simulink model "ROBOT_OK"  (R2021a)
settings: Solver=FixedStepAuto  StartTime=0.0  StopTime=inf  FixedStep=0.001  RelTol=1e-3
model workspace: external: MATLAB File E:\2024\TINH_TOAN_ROBOT_6_DOF\ROBOT_OK_DataFile.m (data not in the file)
values from neighbouring files (symbols this model uses):
  X = Toado(:,1)    [QuydaoK.m]
  Y = Toado(:,2)    [QuydaoK.m]
  Z = Toado(:,3)    [QuydaoK.m]
undefined symbols (not defined in the file or in its folder): smiData
libraries: sm_lib x38, nesl_utility x30, sharedutil x16, sharedtransform x12, dspmtrx3 x12, simulink_extras x8, pid_lib x6, simulink x3
(part 6 of 6)

== matlab function ROBOT_OK/Động Lực Học2/M(q),C(q,dq),g(q)/M,H/W1 ==
  data: w1 input; W output; w2 input; w3 input
function W = fcn(w1,w2,w3)

W = [0    -w3  w2
     w3    0  -w1
    -w2    w1  0];

== matlab function ROBOT_OK/Động Lực Học2/M(q),C(q,dq),g(q)/M,H/W2 ==
  data: w1 input; W output; w2 input; w3 input
function W = fcn(w1,w2,w3)

W = [0    -w3  w2
     w3  0    -w1
    -w2  w1  0];

== matlab function ROBOT_OK/Động Lực Học2/M(q),C(q,dq),g(q)/M,H/W3 ==
  data: w1 input; W output; w2 input; w3 input
function W = fcn(w1,w2,w3)

W = [0    -w3  w2
     w3  0    -w1
    -w2  w1  0];

== matlab function ROBOT_OK/Động Lực Học2/M(q),C(q,dq),g(q)/M,H/W4 ==
  data: w1 input; W output; w2 input; w3 input
function W = fcn(w1,w2,w3)

W = [0    -w3  w2
     w3  0    -w1
    -w2  w1  0];

== matlab function ROBOT_OK/Động Lực Học2/M(q),C(q,dq),g(q)/M,H/W5 ==
  data: w1 input; W output; w2 input; w3 input
function W = fcn(w1,w2,w3)

W = [0    -w3  w2
     w3  0    -w1
    -w2  w1  0];

== matlab function ROBOT_OK/Động Lực Học2/M(q),C(q,dq),g(q)/M,H/W6 ==
  data: w1 input; W output; w2 input; w3 input
function W = fcn(w1,w2,w3)

W = [0    -w3  w2
     w3  0    -w1
    -w2  w1  0];

== matlab function ROBOT_OK/Subsystem2/H_6^0/H_6^5/MATLAB Function ==
  data: R input; H output; p input
function H = fcn(R,p)

H = [R          p
     zeros(1,3) 1];

== matlab function ROBOT_OK/Subsystem2/Jacobian/J_w/J_w_1 ==
  data: R input; J_w output; type input
function J_w = fcn(R,type)

if type==1
    
    J_w=R*[0;0;1];
    
else
    
    J_w=zeros(3,1);
    
end

== matlab function ROBOT_OK/Subsystem2/Jacobian/J_w/J_w_2 ==
  data: R input; J_w output; type input
function J_w = fcn(R,type)

if type==1
    
    J_w=R*[0;0;1];
    
else
    
    J_w=zeros(3,1);
    
end

== matlab function ROBOT_OK/Subsystem2/Jacobian/J_w/J_w_3 ==
  data: R input; J_w output; type input
function J_w = fcn(R,type)

if type==1
    
    J_w=R*[0;0;1];
    
else
    
    J_w=zeros(3,1);
    
end

== matlab function ROBOT_OK/Subsystem2/Jacobian/J_w/J_w_4 ==
  data: R input; J_w output; type input
function J_w = fcn(R,type)

if type==1
    
    J_w=R*[0;0;1];
    
else
    
    J_w=zeros(3,1);
    
end

== matlab function ROBOT_OK/Subsystem2/Jacobian/J_w/J_w_5 ==
  data: R input; J_w output; type input
function J_w = fcn(R,type)

if type==1
    
    J_w=R*[0;0;1];
    
else
    
    J_w=zeros(3,1);
    
end

== matlab function ROBOT_OK/Subsystem2/Jacobian/J_w/J_w_6 ==
  data: R input; J_w output; type input
function J_w = fcn(R,type)

if type==1
    
    J_w=R*[0;0;1];
    
else
    
    J_w=zeros(3,1);
    
end

== matlab function ROBOT_OK/Subsystem2/Jacobian/J_w/v2M_1 ==
  data: v1 input; M output; v2 input
function M = fcn(v1,v2)

M=[v1 v2];

== matlab function ROBOT_OK/Subsystem2/Jacobian/J_w/v2M_2 ==
  data: v1 input; M output; v2 input
function M = fcn(v1,v2)

M=[v1 v2];

== matlab function ROBOT_OK/Subsystem2/Jacobian/J_w/v2M_3 ==
  data: v1 input; M output; v2 input
function M = fcn(v1,v2)

M=[v1 v2];

== matlab function ROBOT_OK/Subsystem2/Jacobian/J_w/v2M_4 ==
  data: v1 input; M output; v2 input
function M = fcn(v1,v2)

M=[v1 v2];

== matlab function ROBOT_OK/Subsystem2/Jacobian/J(q) gen./J_v_1(q)/v2M_2 ==
  data: v1 input; M output; v2 input
function M = fcn(v1,v2)

M=[v1 v2];

== matlab function ROBOT_OK/Subsystem2/Jacobian/J(q) gen./J_v_1(q)/v2M_3 ==
  data: v1 input; M output; v2 input
function M = fcn(v1,v2)

M=[v1 v2];

== matlab function ROBOT_OK/Subsystem2/Jacobian/J(q) gen./J_v_1(q)/v2M_4 ==
  data: v1 input; M output; v2 input
function M = fcn(v1,v2)

M=[v1 v2];

== matlab function ROBOT_OK/Subsystem2/Jacobian/J(q) gen./J_v_1(q)/v2M_5 ==
  data: v1 input; M output; v2 input
function M = fcn(v1,v2)

M=[v1 v2];

== matlab function ROBOT_OK/Subsystem2/Jacobian/J(q) gen./J_v_2(q)/v2M_1 ==
  data: v1 input; M output; v2 input
function M = fcn(v1,v2)

M=[v1 v2];

== matlab function ROBOT_OK/Subsystem2/Jacobian/J(q) gen./J_v_2(q)/v2M_2 ==
  data: v1 input; M output; v2 input
function M = fcn(v1,v2)

M=[v1 v2];

== matlab function ROBOT_OK/Subsystem2/Jacobian/J_v/v2M_1 ==
  data: v1 input; M output; v2 input
function M = fcn(v1,v2)

M=[v1 v2];

== matlab function ROBOT_OK/Subsystem2/Jacobian/J_v/v2M_2 ==
  data: v1 input; M output; v2 input
function M = fcn(v1,v2)

M=[v1 v2];

== matlab function ROBOT_OK/Subsystem2/Jacobian/J_v/v2M_3 ==
  data: v1 input; M output; v2 input
function M = fcn(v1,v2)

M=[v1 v2];

== matlab function ROBOT_OK/Subsystem2/Jacobian/J_v/v2M_4 ==
  data: v1 input; M output; v2 input
function M = fcn(v1,v2)

M=[v1 v2];

== matlab function ROBOT_OK/Subsystem2/Jacobian/J_v/v2M_5 ==
  data: v1 input; M output; v2 input
function M = fcn(v1,v2)

M=[v1 v2];

== matlab function ROBOT_OK/Subsystem2/Jacobian/J_w/v2M_5 ==
  data: v1 input; M output; v2 input
function M = fcn(v1,v2)

M=[v1 v2];

== matlab function ROBOT_OK/Subsystem2/M(q),C(q,dq),g(q)/M,H/MATLAB Function ==
  data: m input; M output; I1 input; I2 input; I3 input; I4 input; I5 input; I6 input; W1 input; W2 input; W3 input; W4 input; W5 input; W6 input; H output
function [M,H] = fcn(m,I1,I2,I3,I4,I5,I6,W1,W2,W3,W4,W5,W6)
%#codegen

M = blkdiag(m(1)*eye(3),m(2)*eye(3),m(3)*eye(3),m(4)*eye(3),m(5)*eye(3),m(6)*eye(3),...
            I1,I2,I3,I4,I5,I6);

H =-blkdiag(zeros(18,18),W1,W2,W3,W4,W5,W6);

== matlab function ROBOT_OK/Subsystem2/M(q),C(q,dq),g(q)/M,H/W1 ==
  data: w1 input; W output; w2 input; w3 input
function W = fcn(w1,w2,w3)

W = [0    -w3  w2
     w3    0  -w1
    -w2    w1  0];

== matlab function ROBOT_OK/Subsystem2/M(q),C(q,dq),g(q)/M,H/W2 ==
  data: w1 input; W output; w2 input; w3 input
function W = fcn(w1,w2,w3)

W = [0    -w3  w2
     w3  0    -w1
    -w2  w1  0];

== matlab function ROBOT_OK/Subsystem2/M(q),C(q,dq),g(q)/M,H/W3 ==
  data: w1 input; W output; w2 input; w3 input
function W = fcn(w1,w2,w3)

W = [0    -w3  w2
     w3  0    -w1
    -w2  w1  0];

== matlab function ROBOT_OK/Subsystem2/M(q),C(q,dq),g(q)/M,H/W4 ==
  data: w1 input; W output; w2 input; w3 input
function W = fcn(w1,w2,w3)

W = [0    -w3  w2
     w3  0    -w1
    -w2  w1  0];

== matlab function ROBOT_OK/Subsystem2/M(q),C(q,dq),g(q)/M,H/W5 ==
  data: w1 input; W output; w2 input; w3 input
function W = fcn(w1,w2,w3)

W = [0    -w3  w2
     w3  0    -w1
    -w2  w1  0];

== matlab function ROBOT_OK/Subsystem2/Jacobian/J(q) gen./J_v_2(q)/v2M_3 ==
  data: v1 input; M output; v2 input
function M = fcn(v1,v2)

M=[v1 v2];

== matlab function ROBOT_OK/Subsystem2/Jacobian/J(q) gen./J_v_2(q)/v2M_4 ==
  data: v1 input; M output; v2 input
function M = fcn(v1,v2)

M=[v1 v2];

== matlab function ROBOT_OK/Subsystem2/Jacobian/J(q) gen./J_v_2(q)/v2M_5 ==
  data: v1 input; M output; v2 input
function M = fcn(v1,v2)

M=[v1 v2];

== matlab function ROBOT_OK/Subsystem2/Jacobian/J(q) gen./J_v_3(q)/v2M_1 ==
  data: v1 input; M output; v2 input
function M = fcn(v1,v2)

M=[v1 v2];

== matlab function ROBOT_OK/Subsystem2/Jacobian/J(q) gen./J_v_3(q)/v2M_2 ==
  data: v1 input; M output; v2 input
function M = fcn(v1,v2)

M=[v1 v2];

== matlab function ROBOT_OK/Subsystem2/Jacobian/J(q) gen./J_v_3(q)/v2M_3 ==
  data: v1 input; M output; v2 input
function M = fcn(v1,v2)

M=[v1 v2];

== matlab function ROBOT_OK/Subsystem2/Jacobian/J(q) gen./J_v_3(q)/v2M_4 ==
  data: v1 input; M output; v2 input
function M = fcn(v1,v2)

M=[v1 v2];

== matlab function ROBOT_OK/Subsystem2/Jacobian/J(q) gen./J_v_3(q)/v2M_5 ==
  data: v1 input; M output; v2 input
function M = fcn(v1,v2)

M=[v1 v2];

== matlab function ROBOT_OK/Subsystem2/Jacobian/J(q) gen./J_v_4(q)/v2M_1 ==
  data: v1 input; M output; v2 input
function M = fcn(v1,v2)

M=[v1 v2];

== matlab function ROBOT_OK/Subsystem2/Jacobian/J(q) gen./J_v_4(q)/v2M_2 ==
  data: v1 input; M output; v2 input
function M = fcn(v1,v2)

M=[v1 v2];

== matlab function ROBOT_OK/Subsystem2/Jacobian/J(q) gen./J_v_4(q)/v2M_3 ==
  data: v1 input; M output; v2 input
function M = fcn(v1,v2)

M=[v1 v2];

== matlab function ROBOT_OK/Subsystem2/Jacobian/J(q) gen./J_v_4(q)/v2M_4 ==
  data: v1 input; M output; v2 input
function M = fcn(v1,v2)

M=[v1 v2];

== matlab function ROBOT_OK/Subsystem2/Jacobian/J(q) gen./J_v_4(q)/v2M_5 ==
  data: v1 input; M output; v2 input
function M = fcn(v1,v2)

M=[v1 v2];

== matlab function ROBOT_OK/Subsystem2/Jacobian/J(q) gen./J_v_5(q)/v2M_1 ==
  data: v1 input; M output; v2 input
function M = fcn(v1,v2)

M=[v1 v2];

== matlab function ROBOT_OK/Subsystem2/Jacobian/J(q) gen./J_v_5(q)/v2M_2 ==
  data: v1 input; M output; v2 input
function M = fcn(v1,v2)

M=[v1 v2];

== matlab function ROBOT_OK/Subsystem2/Jacobian/J(q) gen./J_v_5(q)/v2M_3 ==
  data: v1 input; M output; v2 input
function M = fcn(v1,v2)

M=[v1 v2];

== matlab function ROBOT_OK/Subsystem2/Jacobian/J(q) gen./J_v_5(q)/v2M_4 ==
  data: v1 input; M output; v2 input
function M = fcn(v1,v2)

M=[v1 v2];

== matlab function ROBOT_OK/Subsystem2/Jacobian/J(q) gen./J_v_5(q)/v2M_5 ==
  data: v1 input; M output; v2 input
function M = fcn(v1,v2)

M=[v1 v2];

== matlab function ROBOT_OK/Subsystem2/Jacobian/J(q) gen./MATLAB Function ==
  data: J_w1 input; J_q output; J_w2 input; J_w3 input; J_w4 input; J_w5 input; J_w6 input; J_v1 input; J_v2 input; J_v3 input; J_v4 input; J_v5 input; J_v6 input; R1 input; R2 input; R3 input; R4 input; R5 input; R6 input
function J_q = fcn(J_w1,J_w2,J_w3,J_w4,J_w5,J_w6,J_v1,J_v2,J_v3,J_v4,J_v5,J_v6,R1,R2,R3,R4,R5,R6)


J_q=[J_v1
     J_v2
     J_v3
     J_v4
     J_v5
     J_v6
     R1'*J_w1 zeros(3,5)
     R2'*J_w1 R2'*J_w2 zeros(3,4)
     R3'*J_w1 R3'*J_w2 R3'*J_w3 zeros(3,3)
     R4'*J_w1 R4'*J_w2 R4'*J_w3 R4'*J_w4 zeros(3,2)
     R5'*J_w1 R5'*J_w2 R5'*J_w3 R5'*J_w4 R5'*J_w5 zeros(3,1)
     R6'*J_w1 R6'*J_w2 R6'*J_w3 R6'*J_w4 R6'*J_w5 R6'*J_w6];

== matlab function ROBOT_OK/Subsystem/MATLAB Function1 ==
  data: u input; y1 output; y2 output; y3 output; y4 output; y5 output; y6 output
function [y1,y2,y3,y4,y5,y6]= fcn(u)

y1 = 0*sin(u);
y2 = 0*sin(u);
y3 = 90*sin(u);
y4 = 0*sin(u);
y5 = 90*cos(u);
y6 = 0*sin(u);

% chạy tròn
% y1 = 180*sin(u);
% y2 = 0*sin(u);
% y3 = 0
% y4 = 0*sin(u);
% y5 = 90
% y6 = 90*sin(u);

== matlab function ROBOT_OK/Subsystem2/M(q),C(q,dq),g(q)/M,H/W6 ==
  data: w1 input; W output; w2 input; w3 input
function W = fcn(w1,w2,w3)

W = [0    -w3  w2
     w3  0    -w1
    -w2  w1  0];

== matlab function ROBOT_OK/Động Lực Học2/H_6^0/H_1^0/MATLAB Function ==
  data: R input; H output; p input
function H = fcn(R,p)

H = [R          p
     zeros(1,3) 1];

== matlab function ROBOT_OK/Động Lực Học2/H_6^0/H_2^1/MATLAB Function ==
  data: R input; H output; p input
function H = fcn(R,p)

H = [R          p
     zeros(1,3) 1];

== matlab function ROBOT_OK/Động Lực Học2/H_6^0/H_3^2/MATLAB Function ==
  data: R input; H output; p input
function H = fcn(R,p)

H = [R          p
     zeros(1,3) 1];

== matlab function ROBOT_OK/Dong hoc nghich2/DONG HOC NGHICH ==
  data: P_EE input; the1 output; the2 output; yaw input; pitch input; roll input; the3 output; the4 output; the5 output; the6 output
function [the1,the2,the3,the4,the5,the6] = IK_6DOF(P_EE,yaw,pitch,roll)
%% Thong so cua Robot 6DoF
L2=680; L3=675; L4=282; d1=260; d2=675; d3=173.42;
% A = [0 0 0 0 0 0;0 0 0 0 0 0;0 0 0 0 0 0;0 0 0 0 0 0;0 0 0 0 0 0;0 0 0 0 0 0;0 0 0 0 0 0;0 0 0 0 0 0];
%% Bo nghiem cua loi giai dong hoc nghich
i = 2;
%% Huong cua Robot
r11 = cosd(yaw)*cosd(pitch);
r12 = cosd(yaw)*sind(pitch)*sind(roll) - sind(yaw)*cosd(roll);
r13 = cosd(yaw)*sind(pitch)*cosd(roll) + sind(yaw)*sind(roll);
r21 = sind(yaw)*cosd(pitch);
r22 = sind(yaw)*sind(pitch)*sind(roll) + cosd(yaw)*cosd(roll);
r23 = sind(yaw)*sind(pitch)*cosd(roll) - cosd(yaw)*sind(roll);
r31 = -sind(pitch);
r32 = cosd(pitch)*sind(roll);
r33 = cosd(pitch)*cosd(roll);
Px = P_EE(1) - L4*r13;
Py = P_EE(2) - L4*r23;
Pz = P_EE(3) - L4*r33;
%% Tinh theta1
s1 = real(Py/(sqrt(Px^2+Py^2)));
c1 = real(sqrt(1-s1^2));
t1 = [atan2d(s1,c1);
      atan2d(s1,-c1);];
if (i >= 1 && i <= 4)
    the1 = t1(1);
end
if (i >= 5 && i <= 8)
    the1 = t1(2);
end
% for i1 = 1:8
%     A(i1,1) = the1;
% end
%% Tinh theta3
K = ((Px*cosd(the1)+Py*sind(the1)-d1)^2+(Pz-d2)^2-d3^2-L2^2-L3^2)/(2*L2);
t3=[atan2d(d3,L3) - atan2d(K,sqrt(d3^2+L3^2-K^2));
    atan2d(d3,L3) - atan2d(K,-sqrt(d3^2+L3^2-K^2));];
if (i==1 || i==2 || i==5 || i==6)
    the3 = t3(1);
end
if (i==3 || i==4 || i==7 || i==8)
    the3 = t3(2);
end
% for i3 = 1:8
%     A(i3,3) = the3;
% end
%% Tinh theta2
a3=Px*cosd(the1)+Py*sind(the1)-d1;
b3=Pz-d2;
a11=L3*cosd(the3) + d3*sind(the3);
a12=L2 + d3*cosd(the3) - L3*sind(the3);
a21=d3*cosd(the3) - L3*sind(the3) + L2;
a22=-d3*sind(the3) - L3*cosd(the3);
c2=(a3*a22-b3*a12)/(a11*a22-a21*a12);
s2=(a11*b3-a21*a3)/(a11*a22-a21*a12);
the2 = atan2d(s2,c2);
% for i2 = 1:8
%     A(i2,2) = the2;
% end
%% Tinh theta5
c5= r13*cosd(the2 + the3)*cosd(the1) - r33*sind(the2 + the3) + r23*cosd(the2 + the3)*sind(the1);
s5= sqrt(1-c5^2);
t5=[atan2d(s5,c5);
    atan2d(-s5,c5);];
if (i==1 || i==3 || i==5 || i==7)
    the5 = t5(1);
end
if (i==2 || i==4 || i==6 || i==8)
    the5 = t5(2);
end
% for i5 = 1:8
%     A(i5,5) = the5;
% end
%% Tinh theta4
s4=(r23*cosd(the1) - r13*sind(the1))/sind(the5);
c4=-(r33*cosd(the2 + the3) + r13*sind(the2 + the3)*cosd(the1) + r23*sind(the2 + the3)*sind(the1))/sind(the5);
the4 = atan2d(s4,c4);
% for i4 = 1:8
%     A(i4,4) = the4;
% end
%% Tinh theta6
s6= -(r12*cosd(the2 + the3)*cosd(the1) - r32*sind(the2 + the3) + r22*cosd(the2 + the3)*sind(the1))/sind(the5);
c6=(r11*cosd(the2 + the3)*cosd(the1) - r31*sind(the2 + the3) + r21*cosd(the2 + the3)*sind(the1))/sind(the5);
the6 = atan2d(s6,c6);
% for i6 = 1:8
%     A(i6,6) = the6;
% end
end

== matlab function ROBOT_OK/Dong hoc nghich3/DONG HOC NGHICH ==
  data: P_EE input; the1 output; the2 output; yaw input; pitch input; roll input; the3 output; the4 output; the5 output; the6 output
function [the1,the2,the3,the4,the5,the6] = IK_6DOF(P_EE,yaw,pitch,roll)
%% Thong so cua Robot 6DoF
% L2=270; L3=295; L4=80; d1=75; d2=335; d3=90;
L2=680; L3=675; L4=282; d1=260; d2=675; d3=173.42;
% A = [0 0 0 0 0 0;0 0 0 0 0 0;0 0 0 0 0 0;0 0 0 0 0 0;0 0 0 0 0 0;0 0 0 0 0 0;0 0 0 0 0 0;0 0 0 0 0 0];
%% Bo nghiem cua loi giai dong hoc nghich
i = 2;
%% Huong cua Robot
r11 = cosd(yaw)*cosd(pitch);
r12 = cosd(yaw)*sind(pitch)*sind(roll) - sind(yaw)*cosd(roll);
r13 = cosd(yaw)*sind(pitch)*cosd(roll) + sind(yaw)*sind(roll);
r21 = sind(yaw)*cosd(pitch);
r22 = sind(yaw)*sind(pitch)*sind(roll) + cosd(yaw)*cosd(roll);
r23 = sind(yaw)*sind(pitch)*cosd(roll) - cosd(yaw)*sind(roll);
r31 = -sind(pitch);
r32 = cosd(pitch)*sind(roll);
r33 = cosd(pitch)*cosd(roll);
Px = P_EE(1) - L4*r13;
Py = P_EE(2) - L4*r23;
Pz = P_EE(3) - L4*r33;
%% Tinh theta1
s1 = Py/(sqrt(Px^2+Py^2));
c1 = sqrt(1-s1^2);
t1 = [atan2d(s1,c1);
      atan2d(s1,-c1);];
if (i >= 1 && i <= 4)
    the1 = t1(1);
end
if (i >= 5 && i <= 8)
    the1 = t1(2);
end
% for i1 = 1:8
%     A(i1,1) = the1;
% end
%% Tinh theta3
K = ((Px*cosd(the1)+Py*sind(the1)-d1)^2+(Pz-d2)^2-d3^2-L2^2-L3^2)/(2*L2);
t3=[atan2d(d3,L3) - atan2d(K,sqrt(d3^2+L3^2-K^2));
    atan2d(d3,L3) - atan2d(K,-sqrt(d3^2+L3^2-K^2));];
if (i==1 || i==2 || i==5 || i==6)
    the3 = t3(1);
end
if (i==3 || i==4 || i==7 || i==8)
    the3 = t3(2);
end
% for i3 = 1:8
%     A(i3,3) = the3;
% end
%% Tinh theta2
a3=Px*cosd(the1)+Py*sind(the1)-d1;
b3=Pz-d2;
a11=L3*cosd(the3) + d3*sind(the3);
a12=L2 + d3*cosd(the3) - L3*sind(the3);
a21=d3*cosd(the3) - L3*sind(the3) + L2;
a22=-d3*sind(the3) - L3*cosd(the3);
c2=(a3*a22-b3*a12)/(a11*a22-a21*a12);
s2=(a11*b3-a21*a3)/(a11*a22-a21*a12);
the2 = atan2d(s2,c2);
% for i2 = 1:8
%     A(i2,2) = the2;
% end
%% Tinh theta5
c5= r13*cosd(the2 + the3)*cosd(the1) - r33*sind(the2 + the3) + r23*cosd(the2 + the3)*sind(the1);
s5= sqrt(1-c5^2);
t5=[atan2d(s5,c5);
    atan2d(-s5,c5);];
if (i==1 || i==3 || i==5 || i==7)
    the5 = t5(1);
end
if (i==2 || i==4 || i==6 || i==8)
    the5 = t5(2);
end
% for i5 = 1:8
%     A(i5,5) = the5;
% end
%% Tinh theta4
s4=(r23*cosd(the1) - r13*sind(the1))/sind(the5);
c4=-(r33*cosd(the2 + the3) + r13*sind(the2 + the3)*cosd(the1) + r23*sind(the2 + the3)*sind(the1))/sind(the5);
the4 = atan2d(s4,c4);
% for i4 = 1:8
%     A(i4,4) = the4;
% end
%% Tinh theta6
s6= -(r12*cosd(the2 + the3)*cosd(the1) - r32*sind(the2 + the3) + r22*cosd(the2 + the3)*sind(the1))/sind(the5);
c6=(r11*cosd(the2 + the3)*cosd(the1) - r31*sind(the2 + the3) + r21*cosd(the2 + the3)*sind(the1))/sind(the5);
the6 = atan2d(s6,c6);
% for i6 = 1:8
%     A(i6,6) = the6;
% end
end

== matlab function ROBOT_OK/Dong hoc thuan1/DONG HOC THUAN ==
  data: the1 input; P_EE output; the2 input; the3 input; the4 input; the5 input; the6 input; yaw output; pitch output; roll output
function [P_EE,yaw,pitch,roll]=FK_6DOF(the1,the2,the3,the4,the5,the6)
%% Thong so cua Robot 6DoF
L2=680; L3=675; L4=282; d1=260; d2=675; d3=173.42;
%% Loi giai dong hoc thuan
P_EE = [cosd(the1)*(d1 + L3*cosd(the2 + the3) + d3*sind(the2 + the3) + L2*sind(the2)) + L4*(cosd(the1)*(cosd(the2 + the3)*cosd(the5) - sind(the2 + the3)*cosd(the4)*sind(the5)) - sind(the1)*sind(the4)*sind(the5));
        sind(the1)*(d1 + L3*cosd(the2 + the3) + d3*sind(the2 + the3) + L2*sind(the2)) + L4*(sind(the1)*(cosd(the2 + the3)*cosd(the5) - sind(the2 + the3)*cosd(the4)*sind(the5)) + cosd(the1)*sind(the4)*sind(the5));
        d2 - L3*sind(the2 + the3) + d3*cosd(the2 + the3) + L2*cosd(the2) - L4*(sind(the2 + the3)*cosd(the5) + cosd(the2 + the3)*cosd(the4)*sind(the5));
        1;];
%% Thanh phan huong cua Robot 6DoF
r11= sind(the6)*(cosd(the4)*sind(the1) - sind(the4)*(cosd(the1)*cosd(the2)*sind(the3) + cosd(the1)*cosd(the3)*sind(the2))) + cosd(the6)*(cosd(the5)*(sind(the1)*sind(the4) + cosd(the4)*(cosd(the1)*cosd(the2)*sind(the3) + cosd(the1)*cosd(the3)*sind(the2))) - sind(the5)*(cosd(the1)*sind(the2)*sind(the3) - cosd(the1)*cosd(the2)*cosd(the3)));
r12= cosd(the6)*(cosd(the4)*sind(the1) - sind(the4)*(cosd(the1)*cosd(the2)*sind(the3) + cosd(the1)*cosd(the3)*sind(the2))) - sind(the6)*(cosd(the5)*(sind(the1)*sind(the4) + cosd(the4)*(cosd(the1)*cosd(the2)*sind(the3) + cosd(the1)*cosd(the3)*sind(the2))) - sind(the5)*(cosd(the1)*sind(the2)*sind(the3) - cosd(the1)*cosd(the2)*cosd(the3)));
r13= - sind(the5)*(sind(the1)*sind(the4) + cosd(the4)*(cosd(the1)*cosd(the2)*sind(the3) + cosd(the1)*cosd(the3)*sind(the2))) - cosd(the5)*(cosd(the1)*sind(the2)*sind(the3) - cosd(the1)*cosd(the2)*cosd(the3));
r21= - sind(the6)*(cosd(the1)*cosd(the4) + sind(the4)*(cosd(the2)*sind(the1)*sind(the3) + cosd(the3)*sind(the1)*sind(the2))) - cosd(the6)*(cosd(the5)*(cosd(the1)*sind(the4) - cosd(the4)*(cosd(the2)*sind(the1)*sind(the3) + cosd(the3)*sind(the1)*sind(the2))) + sind(the5)*(sind(the1)*sind(the2)*sind(the3) - cosd(the2)*cosd(the3)*sind(the1)));
r22= sind(the6)*(cosd(the5)*(cosd(the1)*sind(the4) - cosd(the4)*(cosd(the2)*sind(the1)*sind(the3) + cosd(the3)*sind(the1)*sind(the2))) + sind(the5)*(sind(the1)*sind(the2)*sind(the3) - cosd(the2)*cosd(the3)*sind(the1))) - cosd(the6)*(cosd(the1)*cosd(the4) + sind(the4)*(cosd(the2)*sind(the1)*sind(the3) + cosd(the3)*sind(the1)*sind(the2)));
r23= sind(the5)*(cosd(the1)*sind(the4) - cosd(the4)*(cosd(the2)*sind(the1)*sind(the3) + cosd(the3)*sind(the1)*sind(the2))) - cosd(the5)*(sind(the1)*sind(the2)*sind(the3) - cosd(the2)*cosd(the3)*sind(the1));
r31= - cosd(the6)*(sind(the2 + the3)*sind(the5) - cosd(the2 + the3)*cosd(the4)*cosd(the5)) - cosd(the2 + the3)*sind(the4)*sind(the6);
r32= sind(the6)*(sind(the2 + the3)*sind(the5) - cosd(the2 + the3)*cosd(the4)*cosd(the5)) - cosd(the2 + the3)*cosd(the6)*sind(the4);
r33= - sind(the2 + the3)*cosd(the5) - cosd(the2 + the3)*cosd(the4)*sind(the5);
%% Cac goc quay Euler Yaw Pitch Roll
pitch = atan2d(-r31,sqrt(r11^2+r21^2));
yaw = atan2d(r21/cosd(pitch),r11/cosd(pitch));
roll = atan2d(r32/cosd(pitch),r33/cosd(pitch));
end

== matlab function ROBOT_OK/Dong hoc thuan3/DONG HOC THUAN ==
  data: the1 input; P_EE output; the2 input; the3 input; the4 input; the5 input; the6 input; yaw output; pitch output; roll output
function [P_EE,yaw,pitch,roll]=FK_6DOF(the1,the2,the3,the4,the5,the6)
%% Thong so cua Robot 6DoF
L2=680; L3=675; L4=282; d1=260; d2=675; d3=173.42;
%% Loi giai dong hoc thuan
P_EE = [cosd(the1)*(d1 + L3*cosd(the2 + the3) + d3*sind(the2 + the3) + L2*sind(the2)) + L4*(cosd(the1)*(cosd(the2 + the3)*cosd(the5) - sind(the2 + the3)*cosd(the4)*sind(the5)) - sind(the1)*sind(the4)*sind(the5));
        sind(the1)*(d1 + L3*cosd(the2 + the3) + d3*sind(the2 + the3) + L2*sind(the2)) + L4*(sind(the1)*(cosd(the2 + the3)*cosd(the5) - sind(the2 + the3)*cosd(the4)*sind(the5)) + cosd(the1)*sind(the4)*sind(the5));
        d2 - L3*sind(the2 + the3) + d3*cosd(the2 + the3) + L2*cosd(the2) - L4*(sind(the2 + the3)*cosd(the5) + cosd(the2 + the3)*cosd(the4)*sind(the5));
        1;];
%% Thanh phan huong cua Robot 6DoF
r11= sind(the6)*(cosd(the4)*sind(the1) - sind(the4)*(cosd(the1)*cosd(the2)*sind(the3) + cosd(the1)*cosd(the3)*sind(the2))) + cosd(the6)*(cosd(the5)*(sind(the1)*sind(the4) + cosd(the4)*(cosd(the1)*cosd(the2)*sind(the3) + cosd(the1)*cosd(the3)*sind(the2))) - sind(the5)*(cosd(the1)*sind(the2)*sind(the3) - cosd(the1)*cosd(the2)*cosd(the3)));
r12= cosd(the6)*(cosd(the4)*sind(the1) - sind(the4)*(cosd(the1)*cosd(the2)*sind(the3) + cosd(the1)*cosd(the3)*sind(the2))) - sind(the6)*(cosd(the5)*(sind(the1)*sind(the4) + cosd(the4)*(cosd(the1)*cosd(the2)*sind(the3) + cosd(the1)*cosd(the3)*sind(the2))) - sind(the5)*(cosd(the1)*sind(the2)*sind(the3) - cosd(the1)*cosd(the2)*cosd(the3)));
r13= - sind(the5)*(sind(the1)*sind(the4) + cosd(the4)*(cosd(the1)*cosd(the2)*sind(the3) + cosd(the1)*cosd(the3)*sind(the2))) - cosd(the5)*(cosd(the1)*sind(the2)*sind(the3) - cosd(the1)*cosd(the2)*cosd(the3));
r21= - sind(the6)*(cosd(the1)*cosd(the4) + sind(the4)*(cosd(the2)*sind(the1)*sind(the3) + cosd(the3)*sind(the1)*sind(the2))) - cosd(the6)*(cosd(the5)*(cosd(the1)*sind(the4) - cosd(the4)*(cosd(the2)*sind(the1)*sind(the3) + cosd(the3)*sind(the1)*sind(the2))) + sind(the5)*(sind(the1)*sind(the2)*sind(the3) - cosd(the2)*cosd(the3)*sind(the1)));
r22= sind(the6)*(cosd(the5)*(cosd(the1)*sind(the4) - cosd(the4)*(cosd(the2)*sind(the1)*sind(the3) + cosd(the3)*sind(the1)*sind(the2))) + sind(the5)*(sind(the1)*sind(the2)*sind(the3) - cosd(the2)*cosd(the3)*sind(the1))) - cosd(the6)*(cosd(the1)*cosd(the4) + sind(the4)*(cosd(the2)*sind(the1)*sind(the3) + cosd(the3)*sind(the1)*sind(the2)));
r23= sind(the5)*(cosd(the1)*sind(the4) - cosd(the4)*(cosd(the2)*sind(the1)*sind(the3) + cosd(the3)*sind(the1)*sind(the2))) - cosd(the5)*(sind(the1)*sind(the2)*sind(the3) - cosd(the2)*cosd(the3)*sind(the1));
r31= - cosd(the6)*(sind(the2 + the3)*sind(the5) - cosd(the2 + the3)*cosd(the4)*cosd(the5)) - cosd(the2 + the3)*sind(the4)*sind(the6);
r32= sind(the6)*(sind(the2 + the3)*sind(the5) - cosd(the2 + the3)*cosd(the4)*cosd(the5)) - cosd(the2 + the3)*cosd(the6)*sind(the4);
r33= - sind(the2 + the3)*cosd(the5) - cosd(the2 + the3)*cosd(the4)*sind(the5);
%% Cac goc quay Euler Yaw Pitch Roll
pitch = atan2d(-r31,sqrt(r11^2+r21^2));
yaw = atan2d(r21/cosd(pitch),r11/cosd(pitch));
roll = atan2d(r32/cosd(pitch),r33/cosd(pitch));
end

== matlab function ROBOT_OK/MATLAB Function2 ==
  data: t input; Px output; Py output; Pz output
function [Px,Py,Pz] = QUYDAOR(t)
Px=1217; 
Py=200*cos((pi/2)*t);
Pz=1528+200*sin((pi/2)*t);

== matlab function ROBOT_OK/MATLAB Function3 ==
  data: u input; xd output; yd output; zd output
function [xd,yd,zd] = QUYDAOTamgiac(u)
% Tâm của tam giác
    xc = 800;
    yc = 400;
    % Độ dài cạnh của tam giác đều
    a = 500; % Điều chỉnh giá trị này sao cho phù hợp với yêu cầu (không quá 575)
    % Chiều cao của tam giác đều từ trọng tâm đến đỉnh
    h = sqrt(3) / 2 * a; 
    % Tọa độ của ba đỉnh tam giác đều
    x1 = xc;
    y1 = yc + 2 * h / 3; % Đỉnh trên
    x2 = xc - a / 2;
    y2 = yc - h / 3; % Đỉnh dưới bên trái
    x3 = xc + a / 2;
    y3 = yc - h / 3; % Đỉnh dưới bên phải
    % Tính toán các điểm trên quỹ đạo tam giác đều
    u = mod(u, 1); % Đảm bảo u nằm trong khoảng [0, 1]
    if u >= 0 && u < 1/3
        t = u * 3;
        xd = (1 - t) * x1 + t * x2;
        yd = (1 - t) * y1 + t * y2;
    elseif u >= 1/3 && u < 2/3
        t = (u - 1/3) * 3;
        xd = (1 - t) * x2 + t * x3;
        yd = (1 - t) * y2 + t * y3;
    else
        t = (u - 2/3) * 3;
        xd = (1 - t) * x3 + t * x1;
        yd = (1 - t) * y3 + t * y1;
    end
    zd = 1217; % Giữ nguyên giá trị cố định cho zd
end

== matlab function ROBOT_OK/Subsystem2/H_6^0/H_4^3/MATLAB Function ==
  data: R input; H output; p input
function H = fcn(R,p)

H = [R          p
     zeros(1,3) 1];

== matlab function ROBOT_OK/Subsystem/MATLAB Function4 ==
  data: u input; y1 output; y2 output; y3 output; y4 output; y5 output; y6 output
function [y1,y2,y3,y4,y5,y6]= fcn(u)

% y1 = 0*sin(u);
% y2 = 0*sin(u);
% y3 = 90*sin(u);
% y4 = 0*sin(u);
% y5 = 90*cos(u);
% y6 = 0*sin(u);

% chạy tròn
y1 = 180*sin(u);
y2 = 0*sin(u);
y3 = 0
y4 = 0*sin(u);
y5 = 90
y6 = 90*sin(u);

== matlab function ROBOT_OK/Động Lực Học2/H_6^0/H_4^3/MATLAB Function ==
  data: R input; H output; p input
function H = fcn(R,p)

H = [R          p
     zeros(1,3) 1];

== matlab function ROBOT_OK/Động Lực Học2/H_6^0/H_5^4/MATLAB Function ==
  data: R input; H output; p input
function H = fcn(R,p)

H = [R          p
     zeros(1,3) 1];

== matlab function ROBOT_OK/Động Lực Học2/H_6^0/H_6^5/MATLAB Function ==
  data: R input; H output; p input
function H = fcn(R,p)

H = [R          p
     zeros(1,3) 1];

== matlab function ROBOT_OK/Động Lực Học2/Jacobian/J(q) gen./J_v_1(q)/v2M_1 ==
  data: v1 input; M output; v2 input
function M = fcn(v1,v2)

M=[v1 v2];

== matlab function ROBOT_OK/Động Lực Học2/Jacobian/J(q) gen./J_v_1(q)/v2M_2 ==
  data: v1 input; M output; v2 input
function M = fcn(v1,v2)

M=[v1 v2];

== matlab function ROBOT_OK/Động Lực Học2/Jacobian/J(q) gen./J_v_1(q)/v2M_3 ==
  data: v1 input; M output; v2 input
function M = fcn(v1,v2)

M=[v1 v2];

== matlab function ROBOT_OK/Động Lực Học2/Jacobian/J(q) gen./J_v_1(q)/v2M_4 ==
  data: v1 input; M output; v2 input
function M = fcn(v1,v2)

M=[v1 v2];

== matlab function ROBOT_OK/Động Lực Học2/Jacobian/J(q) gen./J_v_1(q)/v2M_5 ==
  data: v1 input; M output; v2 input
function M = fcn(v1,v2)

M=[v1 v2];

== matlab function ROBOT_OK/Động Lực Học2/Jacobian/J(q) gen./J_v_2(q)/v2M_1 ==
  data: v1 input; M output; v2 input
function M = fcn(v1,v2)

M=[v1 v2];

== matlab function ROBOT_OK/Subsystem2/H_6^0/H_3^2/MATLAB Function ==
  data: R input; H output; p input
function H = fcn(R,p)

H = [R          p
     zeros(1,3) 1];

== matlab function ROBOT_OK/Động Lực Học2/Jacobian/J(q) gen./J_v_2(q)/v2M_2 ==
  data: v1 input; M output; v2 input
function M = fcn(v1,v2)

M=[v1 v2];

== matlab function ROBOT_OK/Động Lực Học2/Jacobian/J(q) gen./J_v_2(q)/v2M_3 ==
  data: v1 input; M output; v2 input
function M = fcn(v1,v2)

M=[v1 v2];

== matlab function ROBOT_OK/Động Lực Học2/Jacobian/J(q) gen./J_v_2(q)/v2M_4 ==
  data: v1 input; M output; v2 input
function M = fcn(v1,v2)

M=[v1 v2];

== matlab function ROBOT_OK/Động Lực Học2/Jacobian/J(q) gen./J_v_2(q)/v2M_5 ==
  data: v1 input; M output; v2 input
function M = fcn(v1,v2)

M=[v1 v2];

== matlab function ROBOT_OK/Động Lực Học2/Jacobian/J(q) gen./J_v_3(q)/v2M_1 ==
  data: v1 input; M output; v2 input
function M = fcn(v1,v2)

M=[v1 v2];

== matlab function ROBOT_OK/Động Lực Học2/Jacobian/J(q) gen./J_v_3(q)/v2M_2 ==
  data: v1 input; M output; v2 input
function M = fcn(v1,v2)

M=[v1 v2];

== matlab function ROBOT_OK/Động Lực Học2/Jacobian/J(q) gen./J_v_3(q)/v2M_3 ==
  data: v1 input; M output; v2 input
function M = fcn(v1,v2)

M=[v1 v2];

== matlab function ROBOT_OK/Động Lực Học2/Jacobian/J(q) gen./J_v_3(q)/v2M_4 ==
  data: v1 input; M output; v2 input
function M = fcn(v1,v2)

M=[v1 v2];

== matlab function ROBOT_OK/Động Lực Học2/Jacobian/J(q) gen./J_v_3(q)/v2M_5 ==
  data: v1 input; M output; v2 input
function M = fcn(v1,v2)

M=[v1 v2];

== matlab function ROBOT_OK/Động Lực Học2/Jacobian/J(q) gen./J_v_4(q)/v2M_1 ==
  data: v1 input; M output; v2 input
function M = fcn(v1,v2)

M=[v1 v2];

== matlab function ROBOT_OK/Subsystem2/H_6^0/H_2^1/MATLAB Function ==
  data: R input; H output; p input
function H = fcn(R,p)

H = [R          p
     zeros(1,3) 1];

== matlab function ROBOT_OK/Động Lực Học2/Jacobian/J(q) gen./J_v_4(q)/v2M_2 ==
  data: v1 input; M output; v2 input
function M = fcn(v1,v2)

M=[v1 v2];

== matlab function ROBOT_OK/Động Lực Học2/Jacobian/J(q) gen./J_v_4(q)/v2M_3 ==
  data: v1 input; M output; v2 input
function M = fcn(v1,v2)

M=[v1 v2];

== matlab function ROBOT_OK/Động Lực Học2/Jacobian/J(q) gen./J_v_4(q)/v2M_4 ==
  data: v1 input; M output; v2 input
function M = fcn(v1,v2)

M=[v1 v2];

== matlab function ROBOT_OK/Động Lực Học2/Jacobian/J(q) gen./J_v_4(q)/v2M_5 ==
  data: v1 input; M output; v2 input
function M = fcn(v1,v2)

M=[v1 v2];

== matlab function ROBOT_OK/Động Lực Học2/Jacobian/J(q) gen./J_v_5(q)/v2M_1 ==
  data: v1 input; M output; v2 input
function M = fcn(v1,v2)

M=[v1 v2];

== matlab function ROBOT_OK/Động Lực Học2/Jacobian/J(q) gen./J_v_5(q)/v2M_2 ==
  data: v1 input; M output; v2 input
function M = fcn(v1,v2)

M=[v1 v2];

== matlab function ROBOT_OK/Động Lực Học2/Jacobian/J(q) gen./J_v_5(q)/v2M_3 ==
  data: v1 input; M output; v2 input
function M = fcn(v1,v2)

M=[v1 v2];

== matlab function ROBOT_OK/Động Lực Học2/Jacobian/J(q) gen./J_v_5(q)/v2M_4 ==
  data: v1 input; M output; v2 input
function M = fcn(v1,v2)

M=[v1 v2];

== matlab function ROBOT_OK/Động Lực Học2/Jacobian/J(q) gen./J_v_5(q)/v2M_5 ==
  data: v1 input; M output; v2 input
function M = fcn(v1,v2)

M=[v1 v2];

== matlab function ROBOT_OK/Động Lực Học2/Jacobian/J(q) gen./MATLAB Function ==
  data: J_w1 input; J_q output; J_w2 input; J_w3 input; J_w4 input; J_w5 input; J_w6 input; J_v1 input; J_v2 input; J_v3 input; J_v4 input; J_v5 input; J_v6 input; R1 input; R2 input; R3 input; R4 input; R5 input; R6 input
function J_q = fcn(J_w1,J_w2,J_w3,J_w4,J_w5,J_w6,J_v1,J_v2,J_v3,J_v4,J_v5,J_v6,R1,R2,R3,R4,R5,R6)


J_q=[J_v1
     J_v2
     J_v3
     J_v4
     J_v5
     J_v6
     R1'*J_w1 zeros(3,5)
     R2'*J_w1 R2'*J_w2 zeros(3,4)
     R3'*J_w1 R3'*J_w2 R3'*J_w3 zeros(3,3)
     R4'*J_w1 R4'*J_w2 R4'*J_w3 R4'*J_w4 zeros(3,2)
     R5'*J_w1 R5'*J_w2 R5'*J_w3 R5'*J_w4 R5'*J_w5 zeros(3,1)
     R6'*J_w1 R6'*J_w2 R6'*J_w3 R6'*J_w4 R6'*J_w5 R6'*J_w6];

== matlab function ROBOT_OK/Subsystem2/H_6^0/H_1^0/MATLAB Function ==
  data: R input; H output; p input
function H = fcn(R,p)

H = [R          p
     zeros(1,3) 1];

== matlab function ROBOT_OK/Động Lực Học2/Jacobian/J_v/v2M_1 ==
  data: v1 input; M output; v2 input
function M = fcn(v1,v2)

M=[v1 v2];

== matlab function ROBOT_OK/Động Lực Học2/Jacobian/J_v/v2M_2 ==
  data: v1 input; M output; v2 input
function M = fcn(v1,v2)

M=[v1 v2];

== matlab function ROBOT_OK/Động Lực Học2/Jacobian/J_v/v2M_3 ==
  data: v1 input; M output; v2 input
function M = fcn(v1,v2)

M=[v1 v2];

== matlab function ROBOT_OK/Động Lực Học2/Jacobian/J_v/v2M_4 ==
  data: v1 input; M output; v2 input
function M = fcn(v1,v2)

M=[v1 v2];

== matlab function ROBOT_OK/Động Lực Học2/Jacobian/J_v/v2M_5 ==
  data: v1 input; M output; v2 input
function M = fcn(v1,v2)

M=[v1 v2];

== matlab function ROBOT_OK/Động Lực Học2/Jacobian/J_w/J_w_1 ==
  data: R input; J_w output; type input
function J_w = fcn(R,type)

if type==1
    
    J_w=R*[0;0;1];
    
else
    
    J_w=zeros(3,1);
    
end

== matlab function ROBOT_OK/Động Lực Học2/Jacobian/J_w/J_w_2 ==
  data: R input; J_w output; type input
function J_w = fcn(R,type)

if type==1
    
    J_w=R*[0;0;1];
    
else
    
    J_w=zeros(3,1);
    
end

== matlab function ROBOT_OK/Động Lực Học2/Jacobian/J_w/J_w_3 ==
  data: R input; J_w output; type input
function J_w = fcn(R,type)

if type==1
    
    J_w=R*[0;0;1];
    
else
    
    J_w=zeros(3,1);
    
end

== matlab function ROBOT_OK/Subsystem2/H_6^0/H_5^4/MATLAB Function ==
  data: R input; H output; p input
function H = fcn(R,p)

H = [R          p
     zeros(1,3) 1];

== matlab function ROBOT_OK/Động Lực Học2/Jacobian/J_w/J_w_4 ==
  data: R input; J_w output; type input
function J_w = fcn(R,type)

if type==1
    
    J_w=R*[0;0;1];
    
else
    
    J_w=zeros(3,1);
    
end

== matlab function ROBOT_OK/Động Lực Học2/Jacobian/J_w/J_w_5 ==
  data: R input; J_w output; type input
function J_w = fcn(R,type)

if type==1
    
    J_w=R*[0;0;1];
    
else
    
    J_w=zeros(3,1);
    
end

== matlab function ROBOT_OK/Động Lực Học2/Jacobian/J_w/J_w_6 ==
  data: R input; J_w output; type input
function J_w = fcn(R,type)

if type==1
    
    J_w=R*[0;0;1];
    
else
    
    J_w=zeros(3,1);
    
end

== matlab function ROBOT_OK/Động Lực Học2/Jacobian/J_w/v2M_1 ==
  data: v1 input; M output; v2 input
function M = fcn(v1,v2)

M=[v1 v2];

== matlab function ROBOT_OK/Động Lực Học2/Jacobian/J_w/v2M_2 ==
  data: v1 input; M output; v2 input
function M = fcn(v1,v2)

M=[v1 v2];
